simulink model "StateSpaceIntegralSLXtemplate2016b"  (R2016b)
settings: Solver=VariableStepAuto  StartTime=0.0  StopTime=10.0  RelTol=1e-3
values from neighbouring files (symbols this model uses):
  K = K_amp(1:3)    [plantilla_sscontrol.m]
undefined symbols (not defined in the file or in its folder): kI
settings Model: Creator=aghersin  LastModifiedBy=agher

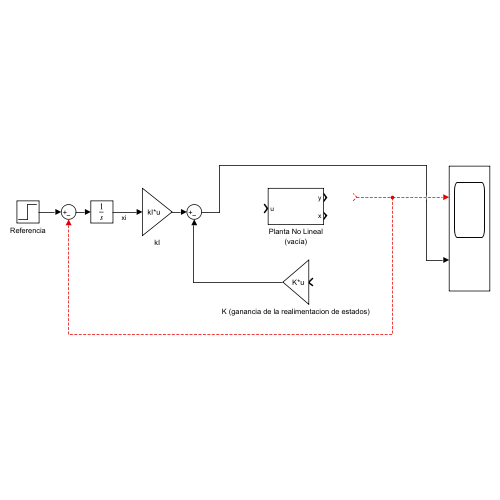
[thumbnail: Simulink's stored preview of the top-level diagram]
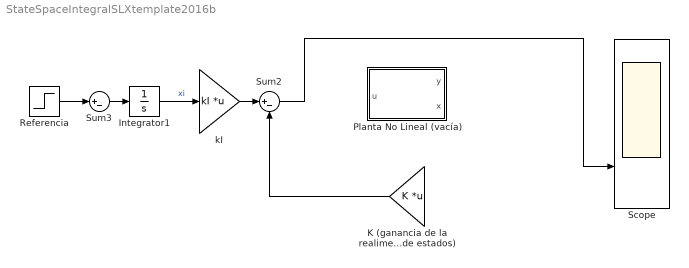
== system StateSpaceIntegralSLXtemplate2016b ==
  Integrator1 : Integrator
  K (ganancia de la realimentacion de estados) : Gain  Gain=K  Multiplication=Matrix(K*u)
  Planta No Lineal (vacía) : Subsystem
  Referencia : Step  SampleTime=0
  Scope : Scope  NumInputPorts=2
  Sum2 : Sum  Inputs=|+-
  Sum3 : Sum  Inputs=|+-
  kI : Gain  Gain=kI  Multiplication=Matrix(K*u)
  wires:
  Referencia/1 -> Sum3/1
  Sum2/1 -> Scope/2
  Sum3/1 -> Integrator1/1
  K (ganancia de la realimentacion de estados)/1 -> Sum2/2
  kI/1 -> Sum2/1
  Integrator1/1 -> kI/1  "xi"
  ? -> Scope/1, Sum3/2

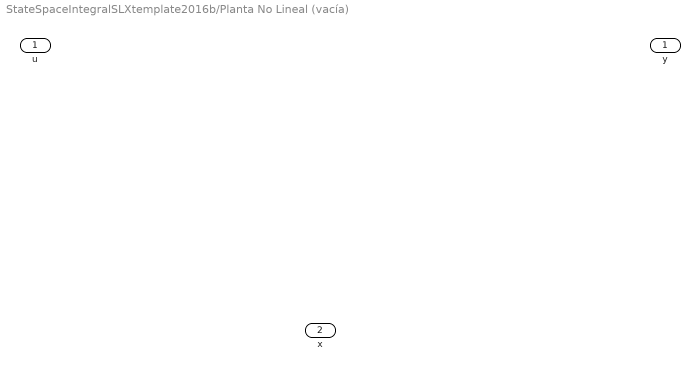
== system StateSpaceIntegralSLXtemplate2016b/Planta No Lineal (vacía) ==
  u : Inport
  y : Outport
  x : Outport  Port=2
